simulink model "TestIMU"  (R2016b)
settings: Solver=VariableStepAuto  StartTime=0.0  StopTime=10.0  RelTol=1e-3
model workspace (MATLAB code in the model file + MAT data in the model file):
  wsHandle = get_param(bdroot, 'modelWorkspace')
  sens = Simulink.Parameter
  sens.Value.rImu_S_m = [0.2413; 0; 0]
  sens.Value.rImu_SB_m = [-0.2413; 0; 0]
  sens.Value.sImu_B_rad = [0; 0; 0]
  sens.Value.T_B2IMU = [1  0  0; 0  1  0; 0  0  1]
  sens.Value.errEnable = 1
  sens.Value.gyroTF_num = 1884.95559215
  sens.Value.gyroTF_den = [1 1884.95559215]
  sens.Value.accelTF_num = 1884.95559215
  sens.Value.accelTF_den = [1 1884.95559215]
  sens.Value.magTF_num = 9676.10537306
  sens.Value.magTF_den = [1 9676.10537306]
  sens.Value.timeDelay_s = 0.001
  sens.Value.gyroScf = [1  0  0; 0  1  0; 0  0  1]
  sens.Value.gyroG = [0  0  0; 0  0  0; 0  0  0]
  sens.Value.gyroBias = [0; 0; 0]
  sens.Value.gyroSigma = [1e-06; 1e-06; 1e-06]
  sens.Value.gyroSeed = [26697; 29681; 4161]
  sens.Value.accelScf = [1  0  0; 0  1  0; 0  0  1]
  sens.Value.accelBias = [0; 0; 0]
  sens.Value.accelSigma = [0.0008; 0.004; 0.004]
  sens.Value.accelSeed = [29929; 20721; 3197]
  sens.Value.magScf = [1  0  0; 0  1  0; 0  0  1]
  sens.Value.magBias = [0; 0; 0]
  sens.Value.magSigma = [150; 150; 80000]
  sens.Value.magSeed = [9126; 17920; 31375]
  sens.Value.timeSample_s = 0.02
  sens.DataType = 'struct'
  sens.Dimensions = [1 1]
  other statements: wsHandle.assignin('sens', AC.Sensors.IMU);
libraries: Sensors_Lib x4
settings Model: ParameterArgumentNames=sens  Creator=rega0051  LastModifiedBy=katiekwiz

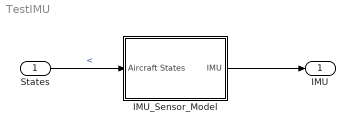
== system TestIMU ==
  "States " : Inport  OutDataTypeStr=Bus: States
  IMU_Sensor_Model : Subsystem  Variant=on  VariantControl=VarIMU_Pass
  " IMU" : Outport  OutDataTypeStr=Bus: IMU
  wires:
  "States "/1 -> IMU_Sensor_Model/1("Aircraft States ")  "<"
  IMU_Sensor_Model/1(" IMU") -> " IMU"/1

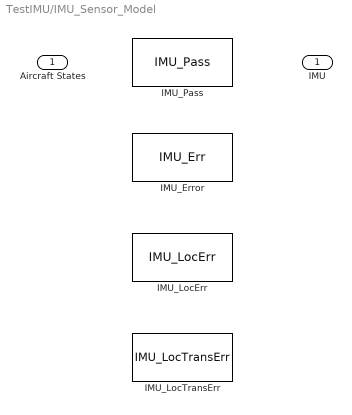
== system TestIMU/IMU_Sensor_Model ==
  "Aircraft States " : Inport
  IMU_Error : Sensors_Lib/IMU Sensor Models/IMU_Err  VariantControl=VarImu_Err
      settings: AttributesFormatString=Variant: %<VariantControl> : %<Variant>
  IMU_LocErr : Sensors_Lib/IMU Sensor Models/IMU_LocErr  VariantControl=VarImu_LocErr
      settings: AttributesFormatString=Variant: %<VariantControl> : %<Variant>
  IMU_LocTransErr : Sensors_Lib/IMU Sensor Models/IMU_LocTransErr  VariantControl=VarImu_LocTransErr
      settings: AttributesFormatString=Variant: %<VariantControl> : %<Variant>
  IMU_Pass : Sensors_Lib/IMU Sensor Models/IMU_Pass  VariantControl=VarImu_Pass
      settings: AttributesFormatString=Variant: %<VariantControl> : %<Variant>
  " IMU" : Outport
